simulink model "ControlloTXRX"  (Simulink 7.5)
settings: Solver=FixedStepDiscrete  StartTime=0.0  StopTime=10.0  FixedStep=0.001  RelTol=1e-3
undefined symbols (not defined in the file or in its folder): DiscIntNeverNeededParam
settings Model: Creator=giada  LastModifiedBy=amministratore
settings OptimizationCC: OptimizeModelRefInitCode=on  LifeSpan=1
settings HardwareCC: ProdBitPerInt=16  ProdIntDivRoundTo=Zero  ProdEndianess=LittleEndian  ProdWordSize=8  ProdHWDeviceType=Atmel->AVR
settings RTWCC: SystemTargetFile=ert_avr.tlc  TemplateMakefile=ert_avr.tmf  Description=AVR Embedded Coder  ProcessScript=ert_avr_make_rtw_hook  CustomSource=ert_main.c  RTWCompilerOptimization=Custom  RTWCustomCompilerOptimizations=atmega169
settings CodeAppCC: IgnoreCustomStorageClasses=off
settings ERTTargetCC: MultiwordLength=2048  SupportAbsoluteTime=off  SupportNonFinite=off  SupportComplex=off  SupportContinuousTime=on  ExtModeMexFile=noextcomm  ERTCustomFileTemplate=example_file_process.tlc  ConvertIfToSwitch=off

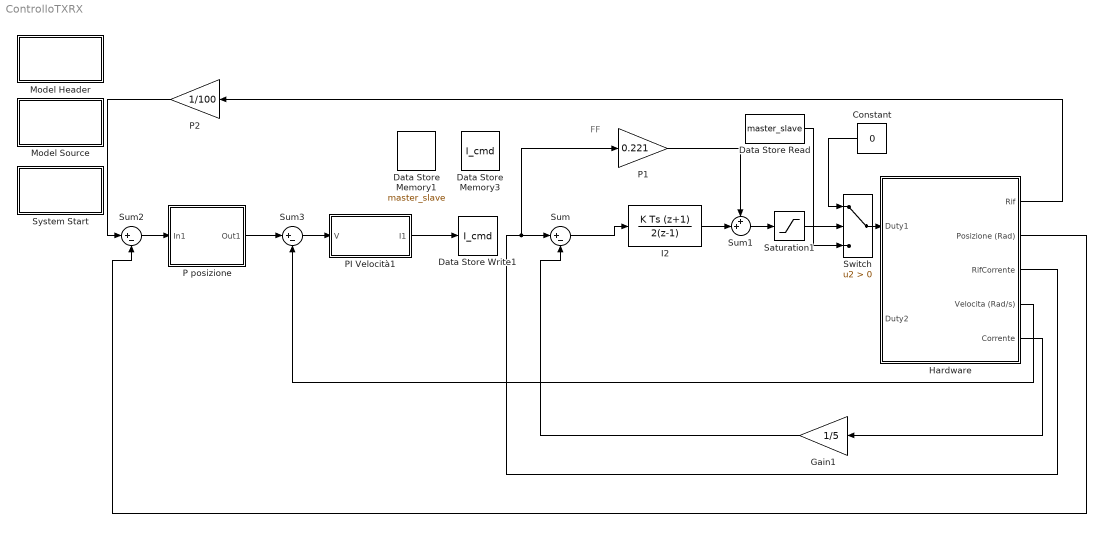
== system ControlloTXRX ==
  note: FF
  Constant : Constant  Value=0  OutDataType=fixdt(1, 16)  OutScaling=2^0
  Data Store Memory1 : DataStoreMemory  DataStoreName=master_slave  ReadBeforeWriteMsg=warning  WriteAfterWriteMsg=warning  WriteAfterReadMsg=warning  DataType=int8  OutDataType=fixdt(1, 16)  OutScaling=2^0  OutDataTypeStr=int8
      settings: RTWStateStorageClass=ExportedGlobal
  Data Store Memory3 : DataStoreMemory  DataStoreName=I_cmd  ReadBeforeWriteMsg=warning  WriteAfterWriteMsg=warning  WriteAfterReadMsg=warning  DataType=single  OutDataType=fixdt(1, 16)  OutScaling=2^0  OutDataTypeStr=single
      settings: RTWStateStorageClass=ExportedGlobal
  Data Store Read : DataStoreRead  DataStoreName=master_slave  SampleTime=0.001
  Data Store Write1 : DataStoreWrite  DataStoreName=I_cmd  SampleTime=0.001
  Gain1 : Gain  Gain=1/5  ParameterDataType=fixdt(1, 16)  ParameterScaling=2^0  OutDataTypeMode=single  OutDataType=fixdt(1, 16)  OutScaling=2^0  OutDataTypeStr=single  SampleTime=0.001
  Hardware : Subsystem
  I2 : DiscreteIntegrator  IntegratorMethod=Integration: Trapezoidal  gainval=1022  SampleTime=0.001  OutDataTypeMode=single  OutDataType=fixdt(1, 16)  OutScaling=2^0  OutDataTypeStr=single  LimitOutput=on  UpperSaturationLimit=0.1  LowerSaturationLimit=0  ICPrevOutput=DiscIntNeverNeededParam  ICPrevScaledInput=DiscIntNeverNeededParam
  Model Header : Subsystem  mask(Model Header){ShowInLibBrowser=0}
      mask prompts: ShowInLibBrowser "Mask Parameter 1:"
      mask help: Add code to the model .h file
      settings: CopyFcn=cccopyfcn(gcb)  OpenFcn=ccopenfcn('Model Header')
      mask Help: eval('feval(''rtwprivate'',''rtwhelpview'',''rtw_model_header_block'')');
      mask Display: disp('Model\nHeader');
  Model Source : Subsystem  mask(Model Source){ShowInLibBrowser=0}
      mask prompts: ShowInLibBrowser "Mask Parameter 1:"
      mask help: Add code to the model .c file
      settings: CopyFcn=cccopyfcn(gcb)  OpenFcn=ccopenfcn('Model Source')
      mask Help: eval('feval(''rtwprivate'',''rtwhelpview'',''rtw_model_source_block'')');
      mask Display: disp('Model\nSource');
  P posizione : Subsystem
  P1 : Gain  Gain=0.221  ParameterDataType=fixdt(1, 16)  ParameterScaling=2^0  OutDataTypeMode=single  OutDataType=fixdt(1, 16)  OutScaling=2^0  OutDataTypeStr=single  SampleTime=0.001
  P2 : Gain  Gain=1/100  ParameterDataType=fixdt(1, 16)  ParameterScaling=2^0  OutDataTypeMode=single  OutDataType=fixdt(1, 16)  OutScaling=2^0  OutDataTypeStr=single  SampleTime=0.001
  PI Velocità1 : Subsystem
  Saturation1 : Saturate  UpperLimit=1  LowerLimit=0  SampleTime=0.001  OutDataTypeMode=single  OutDataType=fixdt(1, 16)  OutScaling=2^0  OutDataTypeStr=single
  Sum : Sum  Inputs=|+-  OutDataType=fixdt(1, 16)  OutScaling=2^0  SampleTime=0.001
  Sum1 : Sum  Inputs=++|  AccumDataTypeStr=single  OutDataType=fixdt(1, 16)  OutScaling=2^0  SampleTime=0.001
  Sum2 : Sum  Inputs=|+-  AccumDataTypeStr=single  OutDataType=fixdt(1, 16)  OutScaling=2^0  SampleTime=0.001
  Sum3 : Sum  Inputs=|+-  AccumDataTypeStr=single  OutDataType=fixdt(1, 16)  OutScaling=2^0  SampleTime=0.001
  Switch : Switch  Criteria=u2 > Threshold  OutDataTypeMode=single  OutDataType=fixdt(1, 16)  OutScaling=2^0  OutDataTypeStr=single
  System Start : Subsystem  mask(System Start){ShowInLibBrowser=0}
      mask prompts: ShowInLibBrowser "Mask Parameter 1:"
      mask help: Add code to a systems Start function
      settings: CopyFcn=cccopyfcn(gcb)  OpenFcn=ccopenfcn('System Start Function')
      mask Help: eval('feval(''rtwprivate'',''rtwhelpview'',''rtw_sys_start_block'')');
      mask Display: disp('System\nStart');
  wires:
  Hardware/5(Corrente) -> Gain1/1
  Sum/1 -> I2/1
  Gain1/1 -> Sum/2
  P1/1 -> Sum1/1
  Sum1/1 -> Saturation1/1
  Hardware/3(RifCorrente) -> Sum/1, P1/1
  Sum2/1 -> P posizione/1(In1)
  Hardware/2(Posizione (Rad)) -> Sum2/2
  I2/1 -> Sum1/2
  Sum3/1 -> PI Velocità1/1(V)
  P2/1 -> Sum2/1
  PI Velocità1/1(I1) -> Data Store Write1/1
  Hardware/4(Velocita (Rad/s)) -> Sum3/2
  Switch/1 -> Hardware/1(Duty1)
  Constant/1 -> Switch/1
  Saturation1/1 -> Switch/3
  Data Store Read/1 -> Switch/2
  Hardware/1(Rif) -> P2/1
  P posizione/1(Out1) -> Sum3/1

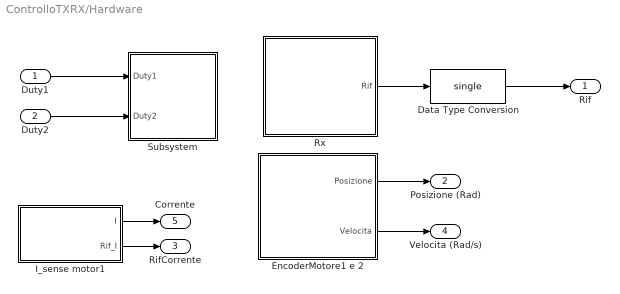
== system ControlloTXRX/Hardware ==
  Duty1 : Inport  OutDataType=fixdt(1, 16)  OutScaling=2^0
  Duty2 : Inport  Port=2  OutDataType=fixdt(1, 16)  OutScaling=2^0
  Data Type Conversion : DataTypeConversion  OutDataTypeMode=single  OutDataType=fixdt(1, 16)  OutScaling=2^0  OutDataTypeStr=single  SampleTime=0.001
  EncoderMotore1 e 2 : Subsystem
  I_sense motor1 : Subsystem
  Rx : Subsystem
  Subsystem : Subsystem
  Rif : Outport  OutDataType=fixdt(1, 16)  OutScaling=2^0
  Posizione (Rad) : Outport  Port=2  OutDataType=fixdt(1, 16)  OutScaling=2^0
  RifCorrente : Outport  Port=3  OutDataType=fixdt(1, 16)  OutScaling=2^0
  Velocita (Rad/s) : Outport  Port=4  OutDataType=fixdt(1, 16)  OutScaling=2^0
  Corrente : Outport  Port=5  OutDataType=fixdt(1, 16)  OutScaling=2^0
  wires:
  Duty1/1 -> Subsystem/1(Duty1)
  Duty2/1 -> Subsystem/2(Duty2)
  EncoderMotore1 e 2/1(Posizione) -> Posizione (Rad)/1
  I_sense motor1/1(I) -> Corrente/1
  Rx/1(Rif) -> Data Type Conversion/1
  EncoderMotore1 e 2/2(Velocita) -> Velocita (Rad/s)/1
  Data Type Conversion/1 -> Rif/1
  I_sense motor1/2(Rif_I) -> RifCorrente/1

== system ControlloTXRX/Model Header ==

== system ControlloTXRX/Model Source ==

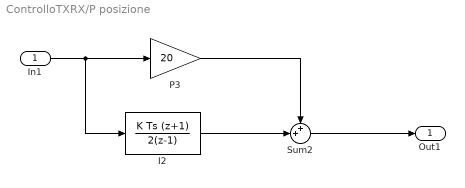
== system ControlloTXRX/P posizione ==
  In1 : Inport
  I2 : DiscreteIntegrator  IntegratorMethod=Integration: Trapezoidal  gainval=50  SampleTime=0.001  OutDataTypeMode=single  OutDataType=fixdt(1, 16)  OutScaling=2^0  OutDataTypeStr=single  LimitOutput=on  UpperSaturationLimit=0.1  LowerSaturationLimit=-0.1  ICPrevOutput=DiscIntNeverNeededParam  ICPrevScaledInput=DiscIntNeverNeededParam
  P3 : Gain  Gain=20  ParameterDataType=fixdt(1, 16)  ParameterScaling=2^0  OutDataTypeMode=single  OutDataType=fixdt(1, 16)  OutScaling=2^0  OutDataTypeStr=single  SampleTime=0.001
  Sum2 : Sum  Inputs=++|  OutDataType=fixdt(1, 16)  OutScaling=2^0  SampleTime=0.001
  Out1 : Outport
  wires:
  In1/1 -> P3/1, I2/1
  Sum2/1 -> Out1/1
  P3/1 -> Sum2/1
  I2/1 -> Sum2/2

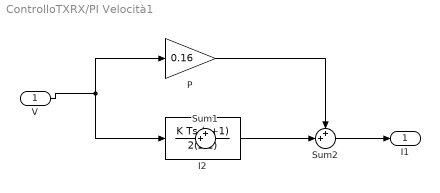
== system ControlloTXRX/PI Velocità1 ==
  V : Inport
  I2 : DiscreteIntegrator  IntegratorMethod=Integration: Trapezoidal  gainval=49  SampleTime=0.001  OutDataTypeMode=single  OutDataType=fixdt(1, 16)  OutScaling=2^0  OutDataTypeStr=single  LimitOutput=on  UpperSaturationLimit=0.1  LowerSaturationLimit=-0.1  ICPrevOutput=DiscIntNeverNeededParam  ICPrevScaledInput=DiscIntNeverNeededParam
  P : Gain  Gain=0.16  ParameterDataType=fixdt(1, 16)  ParameterScaling=2^0  OutDataTypeMode=single  OutDataType=fixdt(1, 16)  OutScaling=2^0  OutDataTypeStr=single  SampleTime=0.001
  Sum1 : Sum  Inputs=++|  OutDataType=fixdt(1, 16)  OutScaling=2^0  SampleTime=0.001
  Sum2 : Sum  Inputs=++|  OutDataType=fixdt(1, 16)  OutScaling=2^0  SampleTime=0.001
  I1 : Outport
  wires:
  Sum2/1 -> I1/1
  P/1 -> Sum2/1
  I2/1 -> Sum2/2
  V/1 -> P/1, I2/1

== system ControlloTXRX/System Start ==

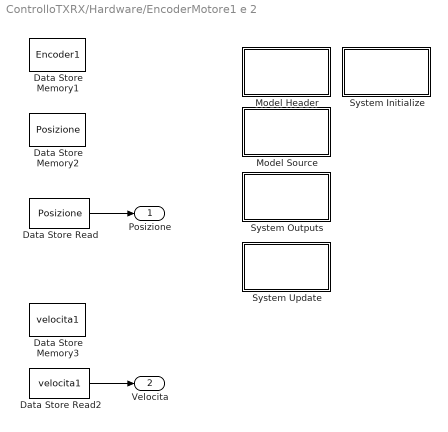
== system ControlloTXRX/Hardware/EncoderMotore1 e 2 ==
  Data Store Memory1 : DataStoreMemory  DataStoreName=Encoder1  ReadBeforeWriteMsg=warning  WriteAfterWriteMsg=warning  WriteAfterReadMsg=warning  DataType=int16  OutDataType=fixdt(1, 16)  OutScaling=2^0  OutDataTypeStr=int16
      settings: RTWStateStorageClass=ExportedGlobal
  Data Store Memory2 : DataStoreMemory  DataStoreName=Posizione  ReadBeforeWriteMsg=warning  WriteAfterWriteMsg=warning  WriteAfterReadMsg=warning  DataType=single  OutDataType=fixdt(1, 16)  OutScaling=2^0  OutDataTypeStr=single
      settings: RTWStateStorageClass=ExportedGlobal
  Data Store Memory3 : DataStoreMemory  DataStoreName=velocita1  ReadBeforeWriteMsg=warning  WriteAfterWriteMsg=warning  WriteAfterReadMsg=warning  DataType=single  OutDataType=fixdt(1, 16)  OutScaling=2^0  OutDataTypeStr=single
      settings: RTWStateStorageClass=ExportedGlobal
  Data Store Read : DataStoreRead  DataStoreName=Posizione  SampleTime=0.001
  Data Store Read2 : DataStoreRead  DataStoreName=velocita1  SampleTime=0.001
  Model Header : Subsystem  mask(Model Header){ShowInLibBrowser=0}
      mask prompts: ShowInLibBrowser "Mask Parameter 1:"
      mask help: Add code to the model .h file
      settings: CopyFcn=cccopyfcn(gcb)  OpenFcn=ccopenfcn('Model Header')
      mask Help: eval('feval(''rtwprivate'',''rtwhelpview'',''rtw_model_header_block'')');
      mask Display: disp('Model\nHeader');
  Model Source : Subsystem  mask(Model Source){ShowInLibBrowser=0}
      mask prompts: ShowInLibBrowser "Mask Parameter 1:"
      mask help: Add code to the model .c file
      settings: CopyFcn=cccopyfcn(gcb)  OpenFcn=ccopenfcn('Model Source')
      mask Help: eval('feval(''rtwprivate'',''rtwhelpview'',''rtw_model_source_block'')');
      mask Display: disp('Model\nSource');
  System Initialize : Subsystem  mask(System Initialize){ShowInLibBrowser=0}
      mask prompts: ShowInLibBrowser "Mask Parameter 1:"
      mask help: Add code to a systems Initialize function
      settings: CopyFcn=cccopyfcn(gcb)  OpenFcn=ccopenfcn('System Initialize Function')
      mask Help: eval('feval(''rtwprivate'',''rtwhelpview'',''rtw_sys_initialize_block'')');
      mask Display: disp('System\nInitialize');
  System Outputs : Subsystem  mask(System Outputs){ShowInLibBrowser=0}
      mask prompts: ShowInLibBrowser "Mask Parameter 1:"
      mask help: Add code to a systems Outputs function
      settings: CopyFcn=cccopyfcn(gcb)  OpenFcn=ccopenfcn('System Outputs Function')
      mask Help: eval('feval(''rtwprivate'',''rtwhelpview'',''rtw_sys_outputs_block'')');
      mask Display: disp('System\nOutputs');
  System Update : Subsystem  mask(System Update){ShowInLibBrowser=0}
      mask prompts: ShowInLibBrowser "Mask Parameter 1:"
      mask help: Add code to a systems Update function
      settings: CopyFcn=cccopyfcn(gcb)  OpenFcn=ccopenfcn('System Update Function')
      mask Help: eval('feval(''rtwprivate'',''rtwhelpview'',''rtw_sys_update_block'')');
      mask Display: disp('System\nUpdate');
  Posizione : Outport  OutDataType=fixdt(1, 16)  OutScaling=2^0
  Velocita : Outport  Port=2  OutDataType=fixdt(1, 16)  OutScaling=2^0
  wires:
  Data Store Read2/1 -> Velocita/1
  Data Store Read/1 -> Posizione/1

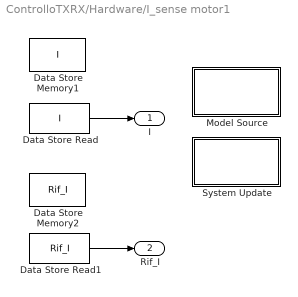
== system ControlloTXRX/Hardware/I_sense motor1 ==
  Data Store Memory1 : DataStoreMemory  DataStoreName=I  ReadBeforeWriteMsg=warning  WriteAfterWriteMsg=warning  WriteAfterReadMsg=warning  DataType=single  OutDataType=fixdt(1, 16)  OutScaling=2^0  OutDataTypeStr=single
      settings: RTWStateStorageClass=ExportedGlobal
  Data Store Memory2 : DataStoreMemory  DataStoreName=Rif_I  ReadBeforeWriteMsg=warning  WriteAfterWriteMsg=warning  WriteAfterReadMsg=warning  DataType=single  OutDataType=fixdt(1, 16)  OutScaling=2^0  OutDataTypeStr=single
      settings: RTWStateStorageClass=ExportedGlobal
  Data Store Read : DataStoreRead  DataStoreName=I  SampleTime=0.001
  Data Store Read1 : DataStoreRead  DataStoreName=Rif_I  SampleTime=0.001
  Model Source : Subsystem  mask(Model Source){ShowInLibBrowser=0}
      mask prompts: ShowInLibBrowser "Mask Parameter 1:"
      mask help: Add code to the model .c file
      settings: CopyFcn=cccopyfcn(gcb)  OpenFcn=ccopenfcn('Model Source')
      mask Help: eval('feval(''rtwprivate'',''rtwhelpview'',''rtw_model_source_block'')');
      mask Display: disp('Model\nSource');
  System Update : Subsystem  mask(System Update){ShowInLibBrowser=0}
      mask prompts: ShowInLibBrowser "Mask Parameter 1:"
      mask help: Add code to a systems Update function
      settings: CopyFcn=cccopyfcn(gcb)  OpenFcn=ccopenfcn('System Update Function')
      mask Help: eval('feval(''rtwprivate'',''rtwhelpview'',''rtw_sys_update_block'')');
      mask Display: disp('System\nUpdate');
  I : Outport  OutDataType=fixdt(1, 16)  OutScaling=2^0
  Rif_I : Outport  Port=2  OutDataType=fixdt(1, 16)  OutScaling=2^0
  wires:
  Data Store Read/1 -> I/1
  Data Store Read1/1 -> Rif_I/1

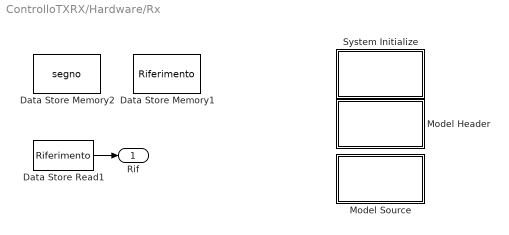
== system ControlloTXRX/Hardware/Rx ==
  Data Store Memory1 : DataStoreMemory  DataStoreName=Riferimento  ReadBeforeWriteMsg=warning  WriteAfterWriteMsg=warning  WriteAfterReadMsg=warning  DataType=int16  OutDataType=fixdt(1, 16)  OutScaling=2^0  OutDataTypeStr=int16
      settings: RTWStateStorageClass=ExportedGlobal
  Data Store Memory2 : DataStoreMemory  DataStoreName=segno  ReadBeforeWriteMsg=warning  WriteAfterWriteMsg=warning  WriteAfterReadMsg=warning  DataType=int8  OutDataType=fixdt(1, 16)  OutScaling=2^0  OutDataTypeStr=int8
      settings: RTWStateStorageClass=ExportedGlobal
  Data Store Read1 : DataStoreRead  DataStoreName=Riferimento  SampleTime=0.001
  Model Header : Subsystem  mask(Model Header){ShowInLibBrowser=0}
      mask prompts: ShowInLibBrowser "Mask Parameter 1:"
      mask help: Add code to the model .h file
      settings: CopyFcn=cccopyfcn(gcb)  OpenFcn=ccopenfcn('Model Header')
      mask Help: eval('feval(''rtwprivate'',''rtwhelpview'',''rtw_model_header_block'')');
      mask Display: disp('Model\nHeader');
  Model Source : Subsystem  mask(Model Source){ShowInLibBrowser=0}
      mask prompts: ShowInLibBrowser "Mask Parameter 1:"
      mask help: Add code to the model .c file
      settings: CopyFcn=cccopyfcn(gcb)  OpenFcn=ccopenfcn('Model Source')
      mask Help: eval('feval(''rtwprivate'',''rtwhelpview'',''rtw_model_source_block'')');
      mask Display: disp('Model\nSource');
  System Initialize : Subsystem  mask(System Initialize){ShowInLibBrowser=0}
      mask prompts: ShowInLibBrowser "Mask Parameter 1:"
      mask help: Add code to a systems Initialize function
      settings: CopyFcn=cccopyfcn(gcb)  OpenFcn=ccopenfcn('System Initialize Function')
      mask Help: eval('feval(''rtwprivate'',''rtwhelpview'',''rtw_sys_initialize_block'')');
      mask Display: disp('System\nInitialize');
  Rif : Outport
  wires:
  Data Store Read1/1 -> Rif/1

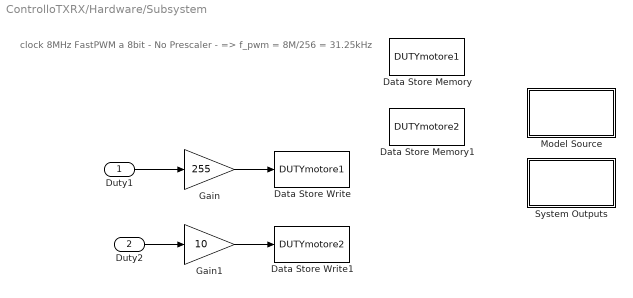
== system ControlloTXRX/Hardware/Subsystem ==
  note: clock 8MHz FastPWM a 8bit - No Prescaler -
      | => f_pwm = 8M/256 = 31.25kHz
  Duty1 : Inport  OutDataType=fixdt(1, 16)  OutScaling=2^0
  Duty2 : Inport  Port=2  OutDataType=fixdt(1, 16)  OutScaling=2^0
  Data Store Memory : DataStoreMemory  DataStoreName=DUTYmotore1  ReadBeforeWriteMsg=warning  WriteAfterWriteMsg=warning  WriteAfterReadMsg=warning  DataType=int16  OutDataType=fixdt(1, 16)  OutScaling=2^0  OutDataTypeStr=int16
      settings: RTWStateStorageClass=ExportedGlobal
  Data Store Memory1 : DataStoreMemory  DataStoreName=DUTYmotore2  ReadBeforeWriteMsg=warning  WriteAfterWriteMsg=warning  WriteAfterReadMsg=warning  DataType=int16  OutDataType=fixdt(1, 16)  OutScaling=2^0  OutDataTypeStr=int16
      settings: RTWStateStorageClass=ExportedGlobal
  Data Store Write : DataStoreWrite  DataStoreName=DUTYmotore1  SampleTime=0.001
  Data Store Write1 : DataStoreWrite  DataStoreName=DUTYmotore2  SampleTime=0.001
  Gain : Gain  Gain=255  ParameterDataType=fixdt(1, 16)  ParameterScaling=2^0  OutDataTypeMode=int16  OutDataType=fixdt(1, 16)  OutScaling=2^0  OutDataTypeStr=int16
  Gain1 : Gain  Gain=10  ParameterDataType=fixdt(1, 16)  ParameterScaling=2^0  OutDataTypeMode=int16  OutDataType=fixdt(1, 16)  OutScaling=2^0  OutDataTypeStr=int16  SampleTime=0.001
  Model Source : Subsystem  mask(Model Source){ShowInLibBrowser=0}
      mask prompts: ShowInLibBrowser "Mask Parameter 1:"
      mask help: Add code to the model .c file
      settings: CopyFcn=cccopyfcn(gcb)  OpenFcn=ccopenfcn('Model Source')
      mask Help: eval('feval(''rtwprivate'',''rtwhelpview'',''rtw_model_source_block'')');
      mask Display: disp('Model\nSource');
  System Outputs : Subsystem  mask(System Outputs){ShowInLibBrowser=0}
      mask prompts: ShowInLibBrowser "Mask Parameter 1:"
      mask help: Add code to a systems Outputs function
      settings: CopyFcn=cccopyfcn(gcb)  OpenFcn=ccopenfcn('System Outputs Function')
      mask Help: eval('feval(''rtwprivate'',''rtwhelpview'',''rtw_sys_outputs_block'')');
      mask Display: disp('System\nOutputs');
  wires:
  Gain/1 -> Data Store Write/1
  Duty1/1 -> Gain/1
  Duty2/1 -> Gain1/1
  Gain1/1 -> Data Store Write1/1

== system ControlloTXRX/Hardware/EncoderMotore1 e 2/Model Header ==

== system ControlloTXRX/Hardware/EncoderMotore1 e 2/Model Source ==

== system ControlloTXRX/Hardware/EncoderMotore1 e 2/System Initialize ==

== system ControlloTXRX/Hardware/EncoderMotore1 e 2/System Outputs ==

== system ControlloTXRX/Hardware/EncoderMotore1 e 2/System Update ==

== system ControlloTXRX/Hardware/I_sense motor1/Model Source ==

== system ControlloTXRX/Hardware/I_sense motor1/System Update ==

== system ControlloTXRX/Hardware/Rx/Model Header ==

== system ControlloTXRX/Hardware/Rx/Model Source ==

== system ControlloTXRX/Hardware/Rx/System Initialize ==

== system ControlloTXRX/Hardware/Subsystem/Model Source ==

== system ControlloTXRX/Hardware/Subsystem/System Outputs ==
